simulink model "Dominant_poles_zeros"  (R2020a)
settings: Solver=VariableStepAuto  StartTime=0.0  StopTime=10.0  RelTol=1e-3
model workspace (MAT data in the model file):
  K = 2000
settings Model: Creator=Kimo Store  LastModifiedBy=Kimo Store

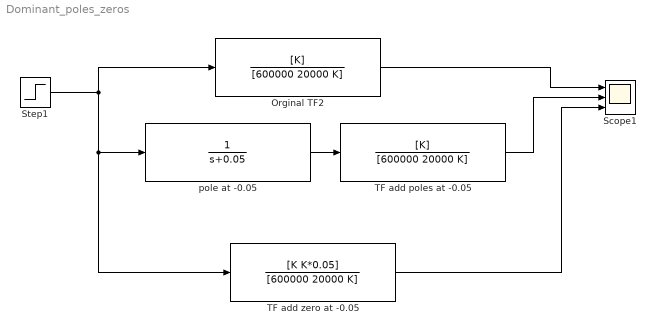
== system Dominant_poles_zeros ==
  Orginal TF2 : TransferFcn  Numerator=[K]  Denominator=[600000 20000 K]
  Scope1 : Scope  NumInputPorts=3
  Step1 : Step  Time=0  SampleTime=0
  TF add poles at -0.05 : TransferFcn  Numerator=[K]  Denominator=[600000 20000 K]
  TF add zero at -0.05 : TransferFcn  Numerator=[K K*0.05]  Denominator=[600000 20000 K]
  pole at -0.05 : TransferFcn  Denominator=[1 0.05]
  wires:
  Orginal TF2/1 -> Scope1/1
  pole at -0.05/1 -> TF add poles at -0.05/1
  TF add zero at -0.05/1 -> Scope1/3
  TF add poles at -0.05/1 -> Scope1/2
  Step1/1 -> Orginal TF2/1, pole at -0.05/1, TF add zero at -0.05/1
